simulink model "Copy_of_R7014E_template_sys"  (R2019a)
settings: Solver=ode5  StartTime=0.0  StopTime=500  RelTol=1e-3  EnableMultiTasking=on
values from neighbouring files (symbols this model uses):
  A = 33    [doubletank.m]    (also in fcn.m; jacobianA.m; kalman_dynamic.m; kalman_dynamic_EKF.m)
  a = 0.16    [doubletank.m]    (also in fcn.m; jacobianA.m; kalman_dynamic.m; kalman_dynamic_EKF.m)
  Amatd = DSYS.A    [kalman_dynamic.m]    (also in kalman_dynamic_EKF.m)
  Bmatd = DSYS.B    [kalman_dynamic.m]    (also in kalman_dynamic_EKF.m)
  Cmatd = DSYS.C    [kalman_dynamic.m]    (also in kalman_dynamic_EKF.m)
  P0 = 1*eye(2)    [kalman_dynamic.m]    (also in kalman_dynamic_EKF.m)
  Ts = 1e-1    (= 0.1)    [kalman_dynamic.m]    (also in kalman_dynamic_EKF.m)
libraries: R7014E_lib x1, simulink x1
settings Model: Creator=wolfgang  LastModifiedBy=lukkar-4
settings Model: ModifiedHistory=|
  | Created an adjusted empty Simulink diagram for the lab assignments
  | in the course R0002E
settings DataIOCC: SaveFormat=Array  SignalLoggingSaveFormat=ModelDataLogs  SaveOutput=off  SignalLogging=off  DSMLogging=off  SaveTime=off  ReturnWorkspaceOutputs=off
settings OptimizationCC: ExpressionDepthLimit=2147483647  LifeSpan=inf
settings DebuggingCC: UnderspecifiedInitializationDetection=Classic  MergeDetectMultiDrivingBlocksExec=none  SolverPrmCheckMsg=warning  FcnCallInpInsideContextMsg=warning  StateNameClashWarn=warning  SFUnexpectedBacktrackingDiag=warning  SFNoUnconditionalDefaultTransitionDiag=warning  SFExecutionAtInitializationDiag=none  ArithmeticOperatorsInVariantConditions=warning
settings HardwareCC: ProdBitPerPointer=32  ProdBitPerSizeT=32  ProdBitPerPtrDiffT=32  ProdLargestAtomicFloat=None  ProdIntDivRoundTo=Undefined  ProdEndianess=Unspecified  ProdWordSize=32  ProdHWDeviceType=32-bit Generic
settings ModelReferenceCC: PropagateSignalLabelsOutOfModel=off
settings SFSimCC: SimUseLocalCustomCode=off
settings RTWCC: RTWUseLocalCustomCode=off
settings CodeAppCC: StateflowObjectComments=on
settings GRTTargetCC: TargetLangStandard=C89/C90 (ANSI)  GeneratePreprocessorConditionals=Disable all
settings ConfigComp: CovMetricSettings=dw  CovHtmlReporting=on  CovSaveCumulativeToWorkspaceVar=on  CovSaveSingleToWorkspaceVar=on  CovExternalEMLEnable=off  CovSFcnEnable=off

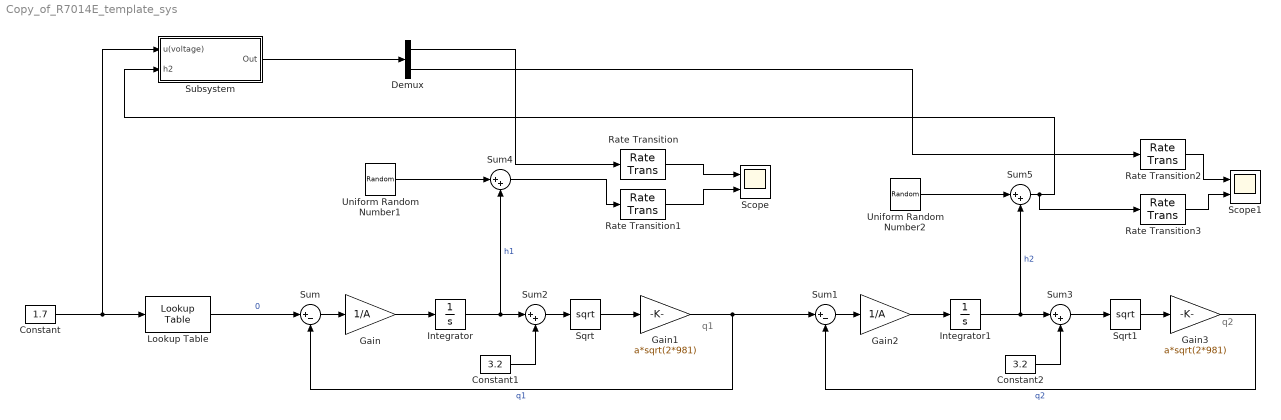
== system Copy_of_R7014E_template_sys ==
  note: q1
  note: q2
  Constant : Constant  Value=1.7  SampleTime=Inf
  Constant1 : Constant  Value=3.2
  Constant2 : Constant  Value=3.2
  Demux : Demux  Outputs=2
  Gain : Gain  Gain=1/A
  Gain1 : Gain  Gain=a*sqrt(2*981)
  Gain2 : Gain  Gain=1/A
  Gain3 : Gain  Gain=a*sqrt(2*981)
  Integrator : Integrator  LimitOutput=on  UpperSaturationLimit=16  LowerSaturationLimit=0
  Integrator1 : Integrator  LimitOutput=on  UpperSaturationLimit=16  LowerSaturationLimit=0
  Lookup Table : R7014E_lib/Lookup Table  x=[0.5,1,1.5,2,2.5,3,3.5,5,8,10]  y=[16.47,20.75,24.52,27.63,30.06,32.49,34.8,40.28,48.24,52.43]
  Rate Transition{,1..3} (4 alike) : RateTransition
  Scope : Scope  NumInputPorts=2
  Scope1 : Scope  NumInputPorts=2
  Sqrt : Sqrt  SaturateOnIntegerOverflow=on
  Sqrt1 : Sqrt  SaturateOnIntegerOverflow=on
  Subsystem : Subsystem
  Sum : Sum  Inputs=|+-
  Sum1 : Sum  Inputs=|+-
  Sum{2..5} (4 alike) : Sum  Inputs=|++
  Uniform Random Number1 : UniformRandomNumber  Minimum=-0.1  Maximum=0.1  SampleTime=Ts
  Uniform Random Number2 : UniformRandomNumber  Minimum=-0.1  Maximum=0.1  SampleTime=Ts
  wires:
  Sum/1 -> Gain/1
  Integrator/1 -> Sum2/1, Sum4/2  "h1"
  Sqrt/1 -> Gain1/1
  Gain1/1 -> Sum1/1, Sum/2  "q1"
  Gain3/1 -> Sum1/2  "q2"
  Sqrt1/1 -> Gain3/1
  Sum1/1 -> Gain2/1
  Lookup Table/1 -> Sum/1  "0"
  Constant/1 -> Subsystem/1(u(voltage)), Lookup Table/1
  Sum2/1 -> Sqrt/1
  Constant1/1 -> Sum2/2
  Constant2/1 -> Sum3/2
  Sum3/1 -> Sqrt1/1
  Uniform Random Number1/1 -> Sum4/1
  Integrator1/1 -> Sum3/1, Sum5/2  "h2"
  Uniform Random Number2/1 -> Sum5/1
  Gain/1 -> Integrator/1
  Gain2/1 -> Integrator1/1
  Sum5/1 -> Rate Transition3/1, Subsystem/2(h2)
  Subsystem/1(Out) -> Demux/1
  Demux/1 -> Rate Transition/1
  Rate Transition/1 -> Scope/1
  Sum4/1 -> Rate Transition1/1
  Rate Transition1/1 -> Scope/2
  Rate Transition2/1 -> Scope1/1
  Rate Transition3/1 -> Scope1/2
  Demux/2 -> Rate Transition2/1

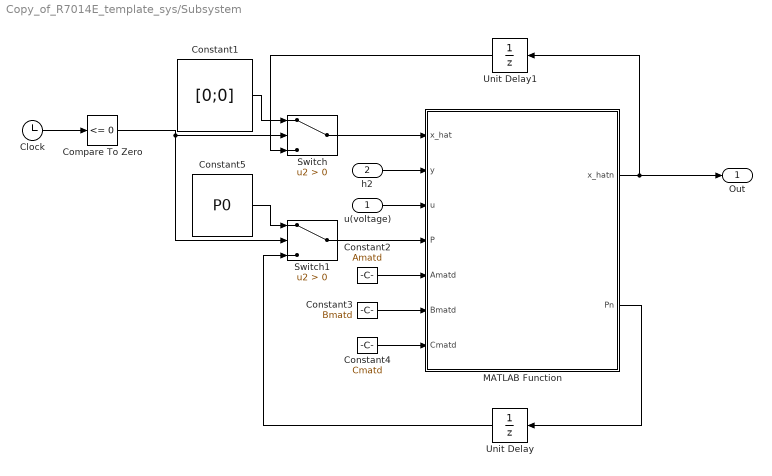
== system Copy_of_R7014E_template_sys/Subsystem ==
  u(voltage) : Inport
  h2 : Inport  Port=2
  Clock : Clock
  Compare To Zero : simulink/Logic and Bit Operations/Compare To Zero  relop=<=  OutDataTypeStr=boolean
  Constant1 : Constant  Value=[0;0]  VectorParams1D=off  SampleTime=Ts
  Constant2 : Constant  Value=Amatd  VectorParams1D=off  SampleTime=Ts
  Constant3 : Constant  Value=Bmatd  VectorParams1D=off  SampleTime=Ts
  Constant4 : Constant  Value=Cmatd  VectorParams1D=off  SampleTime=Ts
  Constant5 : Constant  Value=P0  VectorParams1D=off  SampleTime=Ts
  MATLAB Function : MATLAB Function  TreatAsAtomicUnit=on
  Switch : Switch  Criteria=u2 > Threshold
  Switch1 : Switch  Criteria=u2 > Threshold
  Unit Delay : UnitDelay  SampleTime=Ts  HasFrameUpgradeWarning=on
  Unit Delay1 : UnitDelay  SampleTime=Ts  HasFrameUpgradeWarning=on
  Out : Outport
  wires:
  h2/1 -> MATLAB Function/2(y)
  u(voltage)/1 -> MATLAB Function/3(u)
  Constant2/1 -> MATLAB Function/5(Amatd)
  Constant4/1 -> MATLAB Function/7(Cmatd)
  Constant3/1 -> MATLAB Function/6(Bmatd)
  MATLAB Function/2(Pn) -> Unit Delay/1
  Constant1/1 -> Switch/1
  Unit Delay1/1 -> Switch/3
  Unit Delay/1 -> Switch1/3
  Constant5/1 -> Switch1/1
  Clock/1 -> Compare To Zero/1
  Compare To Zero/1 -> Switch1/2, Switch/2
  Switch1/1 -> MATLAB Function/4(P)
  Switch/1 -> MATLAB Function/1(x_hat)
  MATLAB Function/1(x_hatn) -> Out/1, Unit Delay1/1

== matlab function Copy_of_R7014E_template_sys/Subsystem/MATLAB Function ==
  data: x_hat input; y input; u input; x_hatn output; P input; Pn output; Amatd input; Bmatd input; Cmatd input
function [x_hatn, Pn ] = fcn(x_hat, y, u, P, Amatd, Bmatd, Cmatd)

    Q = 1*eye(2);
    N = 1*eye(2);
    R = 0.1*eye(2);

    x_hatn = Amatd*x_hat + Bmatd*u;
    Pn = Amatd*P*Amatd' + N*Q*N';  

    K = (Pn*Cmatd')\(Cmatd*Pn*Cmatd' + R);
    y_til = y - Cmatd*x_hatn;
    x_hatn = x_hatn + K'*y_til;
   
    Pn = Pn - K'*Cmatd*Pn;
    
end
